simulink model "controller"  (Simulink 7.0)
settings: Solver=ode14x  StartTime=0.0  StopTime=30  FixedStep=0.001  RelTol=1e-3
undefined symbols (not defined in the file or in its folder): DeadMax, DeadMin, Model_626, SaturationMax, SaturationMin, Sensoray
libraries: rtwinlib x3, simulink x3, dsparch4 x1
settings Model: Creator=Student  LastModifiedBy=Student  SimulationMode=external  ExtModeTrigDuration=60000
settings DataIOCC: MaxDataPoints=60000
settings HardwareCC: ProdHWDeviceType=Generic->32-bit Real-Time Simulator  TargetHWDeviceType=32-bit Generic  ProdEqTarget=off
settings RTWCC: SystemTargetFile=rtwin.tlc  TemplateMakefile=rtwin.tmf  Description=Real-Time Windows Target  ProcessScript=rtwin_make_rtw_hook
settings RTWinTargetCC: GenFloatMathFcnCalls=ANSI_C  ModelReferenceCompliant=off  CompOptLevelCompliant=off  PortableWordSizes=off  CCOptimize=on

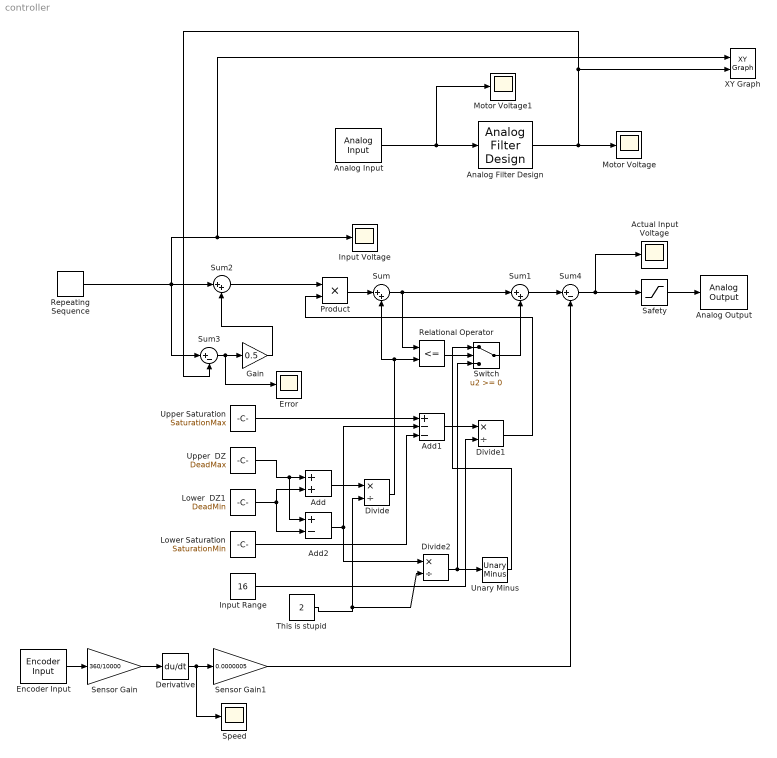
== system controller ==
  Actual Input Voltage : Scope
      settings: TimeRange=60  YMin=-9  YMax=9  SaveName=position5  DataFormat=Array  MaxDataPoints=60000
  Add : Sum  OutDataType=sfix(16)  OutScaling=2^-10
  Add1 : Sum  Inputs=+--  OutDataType=sfix(16)  OutScaling=2^-10
  Add2 : Sum  Inputs=+-  OutDataType=sfix(16)  OutScaling=2^-10
  Analog Filter Design : dsparch4/Analog Filter Design  method=Butterworth  filttype=Lowpass  N=10  Wlo=12  Whi=80  Rp=2  Rs=40
  Analog Input : rtwinlib/Analog Input  SampleTime=0.001  DrvName=Sensoray/Model_626  DrvAddress=4294967295  DrvOptions=zeros(1,0)  Channels=1  RangeMode=1  VoltRange=1  DataType=1
      settings: AttributesFormatString=Sensoray\nModel 626 [auto]
  Analog Output : rtwinlib/Analog Output  SampleTime=0.001  DrvName=Sensoray/Model_626  DrvAddress=4294967295  DrvOptions=zeros(1,0)  Channels=1  RangeMode=1  VoltRange=1  InitialValue=0  FinalValue=0
      settings: AttributesFormatString=Sensoray\nModel 626 [auto]
  Derivative : Derivative
  Divide : Product  Inputs=*/  OutDataType=sfix(16)  OutScaling=2^-10
  Divide1 : Product  Inputs=*/  OutDataType=sfix(16)  OutScaling=2^-10
  Divide2 : Product  Inputs=*/  OutDataType=sfix(16)  OutScaling=2^-10
  Encoder Input : rtwinlib/Encoder Input  SampleTime=0.001  DrvName=Sensoray/Model_626  DrvAddress=4294967295  DrvOptions=zeros(1,0)  Channels=[4]  QuadMode=3  IndexPulse=2  InputFilter=inf  DataType=1
      settings: AttributesFormatString=Sensoray\nModel 626 [auto]
  Error : Scope
      settings: TimeRange=30  YMin=-8  YMax=3  SaveName=position7  DataFormat=Array  MaxDataPoints=60000
  Gain : Gain  Gain=0.5  ParameterDataType=sfix(16)  ParameterScaling=2^0  OutDataType=sfix(16)  OutScaling=2^0
  Input Range : Constant  Value=16  OutDataType=sfix(16)  OutScaling=2^0
  Input Voltage : Scope
      settings: TimeRange=60  YMin=-9  YMax=9  SaveName=position4  DataFormat=Array  MaxDataPoints=60000
  Lower  DZ1 : Constant  Value=DeadMin  OutDataType=sfix(16)  OutScaling=2^0
  Lower Saturation : Constant  Value=SaturationMin  OutDataType=sfix(16)  OutScaling=2^0
  Motor Voltage : Scope
      settings: TimeRange=60  YMin=-8.5  YMax=0.5  SaveName=position1  DataFormat=Array  MaxDataPoints=60000
  Motor Voltage1 : Scope
      settings: TimeRange=60  YMin=-9  YMax=9  SaveName=position6  DataFormat=Array  MaxDataPoints=60000
  Product : Product  OutDataType=sfix(16)  OutScaling=2^0  RndMeth=Zero
  Relational Operator : RelationalOperator  Operator=<=  LogicOutDataTypeMode=boolean
  Repeating Sequence : simulink/Sources/Repeating Sequence  SystemSampleTime=-1  rep_seq_t=[0 30]  rep_seq_y=[-8 8]
  Safety : Saturate  UpperLimit=5  LowerLimit=0.1  SampleTime=0.001  OutDataType=sfix(16)  OutScaling=2^0
  Sensor Gain : Gain  Gain=360/10000  ParameterDataType=sfix(16)  ParameterScaling=2^0  OutDataType=sfix(16)  OutScaling=2^0
  Sensor Gain1 : Gain  Gain=0.0000005  ParameterDataType=sfix(16)  ParameterScaling=2^0  OutDataType=sfix(16)  OutScaling=2^0
  Speed : Scope
      settings: TimeRange=60  YMin=-9  YMax=9  SaveName=position  DataFormat=Array  MaxDataPoints=60000
  Sum : Sum  Inputs=|++  OutDataType=sfix(16)  OutScaling=2^0
  Sum1 : Sum  Inputs=|++  OutDataType=sfix(16)  OutScaling=2^0
  Sum2 : Sum  Inputs=|++  OutDataType=sfix(16)  OutScaling=2^0
  Sum3 : Sum  Inputs=|+-  OutDataType=sfix(16)  OutScaling=2^0
  Sum4 : Sum  Inputs=|+-  OutDataType=sfix(16)  OutScaling=2^0
  Switch : Switch  OutDataType=sfix(16)  OutScaling=2^0
  This is stupid : Constant  Value=2  OutDataType=sfix(16)  OutScaling=2^0
  Unary Minus : simulink/Math Operations/Unary Minus  DoSatur=off
  Upper  DZ : Constant  Value=DeadMax  OutDataType=sfix(16)  OutScaling=2^0
  Upper Saturation : Constant  Value=SaturationMax  OutDataType=sfix(16)  OutScaling=2^0
  XY Graph : simulink/Sinks/XY Graph  SystemSampleTime=-1  xmin=-8  xmax=8  ymin=-8  ymax=8  st=-1
  wires:
  Analog Input/1 -> Analog Filter Design/1, Motor Voltage1/1
  Safety/1 -> Analog Output/1
  Analog Filter Design/1 -> Motor Voltage/1, XY Graph/2, Sum3/2
  Upper  DZ/1 -> Add/1, Add2/1
  Lower  DZ1/1 -> Add/2, Add2/2
  Add/1 -> Divide/1
  This is stupid/1 -> Divide/2, Divide2/2
  Upper Saturation/1 -> Add1/1
  Lower Saturation/1 -> Add1/3
  Input Range/1 -> Divide1/2
  Add1/1 -> Divide1/1
  Divide1/1 -> Product/2
  Product/1 -> Sum/1
  Divide/1 -> Sum/2, Relational Operator/2
  Relational Operator/1 -> Switch/2
  Add2/1 -> Divide2/1, Add1/2
  Sum/1 -> Relational Operator/1, Sum1/1
  Divide2/1 -> Switch/3, Unary Minus/1
  Unary Minus/1 -> Switch/1
  Switch/1 -> Sum1/2
  Repeating Sequence/1 -> XY Graph/1, Input Voltage/1, Sum2/1, Sum3/1
  Sum3/1 -> Gain/1, Error/1
  Gain/1 -> Sum2/2
  Encoder Input/1 -> Sensor Gain/1
  Sensor Gain/1 -> Derivative/1
  Derivative/1 -> Speed/1, Sensor Gain1/1
  Sum2/1 -> Product/1
  Sum1/1 -> Sum4/1
  Sum4/1 -> Safety/1, Actual Input Voltage/1
  Sensor Gain1/1 -> Sum4/2
